simulink model "TBRe19_ECU_SequentialTests"  (R2017b)
settings: Solver=FixedStepDiscrete  StartTime=0.0  StopTime=inf  FixedStep=0.0001  RelTol=1e-3
PostLoadFcn:
  | model_init();
libraries: simulink x28
(part 19 of 22)

== system TBRe19_ECU_SequentialTests/RTDandStateMachine/Comms_And_Data_Acquisition_Layer/Hardwired_Inputs_2019/BMS ==
  DigitalInput1 : S-Function  FunctionName=NsiIo_DigitalInput  Parameters=channel,is_trigger,typeof_trigger,is_wakeup,wakeup_level  SFunctionDeploymentMode=off  EnableBusSupport=off  mask(MUXlink I/O Digital Input){channel=16, is_trigger=off, typeof_trigger=Either, is_wakeup=off, wakeup_level=Low level}
      mask prompts: channel "Channel ?"; is_trigger "Trigger ?"; typeof_trigger "Type of Trigger ?"; is_wakeup "Wake-up ?"; wakeup_level "Wake-up level ?"
      mask help: Read digital input from I/O channel.
      mask init:
      | NsiIo_DigitalInput_InitializationFcn();
      settings: OpenFcn=NsiIo_DigitalInput_OpenFcn();
      mask Help:
      | eval('block=get_param(gcb, ''RTWdata'');')
      | web([docroot '\toolbox\MUXlink\html\blocks/' block.MUXlink_BlockType '.html'])
      mask Callback channel: NsiIo_DigitalInput_ApplyFcn(1);
      mask Callback is_trigger: NsiIo_DigitalInput_ApplyFcn(2);
      mask TypeOptions typeof_trigger: Rising | Falling | Either
      mask Callback typeof_trigger: NsiIo_DigitalInput_ApplyFcn(3);
      mask Callback is_wakeup: NsiIo_DigitalInput_ApplyFcn(4);
      mask TypeOptions wakeup_level: Low level | High level
      mask Callback wakeup_level: NsiIo_DigitalInput_ApplyFcn(5);
      mask Display: image(imread('nsi.bmp'));text(0.5, 0.2, 'DigitalInput_16', 'horizontalAlignment', 'center', 'verticalAlignment', 'base');plot([0.05 0.05 0.05 0.05 0.05 0.05 0.05 0.05 0.05 0.05]);port_label('output', 1, 'Battery : H2');
  DigitalInput2 : S-Function  FunctionName=NsiIo_DigitalInput  Parameters=channel,is_trigger,typeof_trigger,is_wakeup,wakeup_level  SFunctionDeploymentMode=off  EnableBusSupport=off  mask(MUXlink I/O Digital Input){channel=17, is_trigger=off, typeof_trigger=Either, is_wakeup=off, wakeup_level=Low level}
      mask prompts: channel "Channel ?"; is_trigger "Trigger ?"; typeof_trigger "Type of Trigger ?"; is_wakeup "Wake-up ?"; wakeup_level "Wake-up level ?"
      mask help: Read digital input from I/O channel.
      mask init:
      | NsiIo_DigitalInput_InitializationFcn();
      settings: OpenFcn=NsiIo_DigitalInput_OpenFcn();
      mask Help:
      | eval('block=get_param(gcb, ''RTWdata'');')
      | web([docroot '\toolbox\MUXlink\html\blocks/' block.MUXlink_BlockType '.html'])
      mask Callback channel: NsiIo_DigitalInput_ApplyFcn(1);
      mask Callback is_trigger: NsiIo_DigitalInput_ApplyFcn(2);
      mask TypeOptions typeof_trigger: Rising | Falling | Either
      mask Callback typeof_trigger: NsiIo_DigitalInput_ApplyFcn(3);
      mask Callback is_wakeup: NsiIo_DigitalInput_ApplyFcn(4);
      mask TypeOptions wakeup_level: Low level | High level
      mask Callback wakeup_level: NsiIo_DigitalInput_ApplyFcn(5);
      mask Display: image(imread('nsi.bmp'));text(0.5, 0.2, 'DigitalInput_17', 'horizontalAlignment', 'center', 'verticalAlignment', 'base');plot([0.05 0.05 0.05 0.05 0.05 0.05 0.05 0.05 0.05 0.05]);port_label('output', 1, 'Battery : H3');
  DigitalInput6 : S-Function  FunctionName=NsiIo_DigitalInput  Parameters=channel,is_trigger,typeof_trigger,is_wakeup,wakeup_level  SFunctionDeploymentMode=off  EnableBusSupport=off  mask(MUXlink I/O Digital Input){channel=18, is_trigger=off, typeof_trigger=Either, is_wakeup=off, wakeup_level=Low level}
      mask prompts: channel "Channel ?"; is_trigger "Trigger ?"; typeof_trigger "Type of Trigger ?"; is_wakeup "Wake-up ?"; wakeup_level "Wake-up level ?"
      mask help: Read digital input from I/O channel.
      mask init:
      | NsiIo_DigitalInput_InitializationFcn();
      settings: OpenFcn=NsiIo_DigitalInput_OpenFcn();
      mask Help:
      | eval('block=get_param(gcb, ''RTWdata'');')
      | web([docroot '\toolbox\MUXlink\html\blocks/' block.MUXlink_BlockType '.html'])
      mask Callback channel: NsiIo_DigitalInput_ApplyFcn(1);
      mask Callback is_trigger: NsiIo_DigitalInput_ApplyFcn(2);
      mask TypeOptions typeof_trigger: Rising | Falling | Either
      mask Callback typeof_trigger: NsiIo_DigitalInput_ApplyFcn(3);
      mask Callback is_wakeup: NsiIo_DigitalInput_ApplyFcn(4);
      mask TypeOptions wakeup_level: Low level | High level
      mask Callback wakeup_level: NsiIo_DigitalInput_ApplyFcn(5);
      mask Display: image(imread('nsi.bmp'));text(0.5, 0.2, 'DigitalInput_18', 'horizontalAlignment', 'center', 'verticalAlignment', 'base');plot([0.05 0.05 0.05 0.05 0.05 0.05 0.05 0.05 0.05 0.05]);port_label('output', 1, 'Battery : H4');
  BMS_Multi1 : Outport
  BMS_Multi2 : Outport  Port=2
  BMS_ChargeEnable : Outport  Port=3
  wires:
  DigitalInput6/1 -> BMS_Multi1/1  "BMS_Multi1"
  DigitalInput2/1 -> BMS_ChargeEnable/1  "BMS_ChargeEnable"
  DigitalInput1/1 -> BMS_Multi2/1  "BMS_Multi2"

== system TBRe19_ECU_SequentialTests/RTDandStateMachine/Comms_And_Data_Acquisition_Layer/Hardwired_Inputs_2019/Buttons ==
  DigitalInput1 : S-Function  FunctionName=NsiIo_DigitalInput  Parameters=channel,is_trigger,typeof_trigger,is_wakeup,wakeup_level  SFunctionDeploymentMode=off  EnableBusSupport=off  mask(MUXlink I/O Digital Input){channel=5, is_trigger=off, typeof_trigger=Either, is_wakeup=off, wakeup_level=Low level}
      mask prompts: channel "Channel ?"; is_trigger "Trigger ?"; typeof_trigger "Type of Trigger ?"; is_wakeup "Wake-up ?"; wakeup_level "Wake-up level ?"
      mask help: Read digital input from I/O channel.
      mask init:
      | NsiIo_DigitalInput_InitializationFcn();
      settings: OpenFcn=NsiIo_DigitalInput_OpenFcn();
      mask Help:
      | eval('block=get_param(gcb, ''RTWdata'');')
      | web([docroot '\toolbox\MUXlink\html\blocks/' block.MUXlink_BlockType '.html'])
      mask Callback channel: NsiIo_DigitalInput_ApplyFcn(1);
      mask Callback is_trigger: NsiIo_DigitalInput_ApplyFcn(2);
      mask TypeOptions typeof_trigger: Rising | Falling | Either
      mask Callback typeof_trigger: NsiIo_DigitalInput_ApplyFcn(3);
      mask Callback is_wakeup: NsiIo_DigitalInput_ApplyFcn(4);
      mask TypeOptions wakeup_level: Low level | High level
      mask Callback wakeup_level: NsiIo_DigitalInput_ApplyFcn(5);
      mask Display: image(imread('nsi.bmp'));text(0.5, 0.2, 'DigitalInput_5', 'horizontalAlignment', 'center', 'verticalAlignment', 'base');plot([0.05 0.05 0.05 0.05 0.05 0.05 0.05 0.05 0.05 0.05]);port_label('output', 1, 'Ground : B1');
  DigitalInput2 : S-Function  FunctionName=NsiIo_DigitalInput  Parameters=channel,is_trigger,typeof_trigger,is_wakeup,wakeup_level  SFunctionDeploymentMode=off  EnableBusSupport=off  mask(MUXlink I/O Digital Input){channel=8, is_trigger=off, typeof_trigger=Either, is_wakeup=off, wakeup_level=Low level}
      mask prompts: channel "Channel ?"; is_trigger "Trigger ?"; typeof_trigger "Type of Trigger ?"; is_wakeup "Wake-up ?"; wakeup_level "Wake-up level ?"
      mask help: Read digital input from I/O channel.
      mask init:
      | NsiIo_DigitalInput_InitializationFcn();
      settings: OpenFcn=NsiIo_DigitalInput_OpenFcn();
      mask Help:
      | eval('block=get_param(gcb, ''RTWdata'');')
      | web([docroot '\toolbox\MUXlink\html\blocks/' block.MUXlink_BlockType '.html'])
      mask Callback channel: NsiIo_DigitalInput_ApplyFcn(1);
      mask Callback is_trigger: NsiIo_DigitalInput_ApplyFcn(2);
      mask TypeOptions typeof_trigger: Rising | Falling | Either
      mask Callback typeof_trigger: NsiIo_DigitalInput_ApplyFcn(3);
      mask Callback is_wakeup: NsiIo_DigitalInput_ApplyFcn(4);
      mask TypeOptions wakeup_level: Low level | High level
      mask Callback wakeup_level: NsiIo_DigitalInput_ApplyFcn(5);
      mask Display: image(imread('nsi.bmp'));text(0.5, 0.2, 'DigitalInput_8', 'horizontalAlignment', 'center', 'verticalAlignment', 'base');plot([0.05 0.05 0.05 0.05 0.05 0.05 0.05 0.05 0.05 0.05]);port_label('output', 1, 'Ground : B4');
  DigitalInput3 : S-Function  FunctionName=NsiIo_DigitalInput  Parameters=channel,is_trigger,typeof_trigger,is_wakeup,wakeup_level  SFunctionDeploymentMode=off  EnableBusSupport=off  mask(MUXlink I/O Digital Input){channel=6, is_trigger=off, typeof_trigger=Either, is_wakeup=off, wakeup_level=Low level}
      mask prompts: channel "Channel ?"; is_trigger "Trigger ?"; typeof_trigger "Type of Trigger ?"; is_wakeup "Wake-up ?"; wakeup_level "Wake-up level ?"
      mask help: Read digital input from I/O channel.
      mask init:
      | NsiIo_DigitalInput_InitializationFcn();
      settings: OpenFcn=NsiIo_DigitalInput_OpenFcn();
      mask Help:
      | eval('block=get_param(gcb, ''RTWdata'');')
      | web([docroot '\toolbox\MUXlink\html\blocks/' block.MUXlink_BlockType '.html'])
      mask Callback channel: NsiIo_DigitalInput_ApplyFcn(1);
      mask Callback is_trigger: NsiIo_DigitalInput_ApplyFcn(2);
      mask TypeOptions typeof_trigger: Rising | Falling | Either
      mask Callback typeof_trigger: NsiIo_DigitalInput_ApplyFcn(3);
      mask Callback is_wakeup: NsiIo_DigitalInput_ApplyFcn(4);
      mask TypeOptions wakeup_level: Low level | High level
      mask Callback wakeup_level: NsiIo_DigitalInput_ApplyFcn(5);
      mask Display: image(imread('nsi.bmp'));text(0.5, 0.2, 'DigitalInput_6', 'horizontalAlignment', 'center', 'verticalAlignment', 'base');plot([0.05 0.05 0.05 0.05 0.05 0.05 0.05 0.05 0.05 0.05]);port_label('output', 1, 'Ground : B2');
  DigitalInput4 : S-Function  FunctionName=NsiIo_DigitalInput  Parameters=channel,is_trigger,typeof_trigger,is_wakeup,wakeup_level  SFunctionDeploymentMode=off  EnableBusSupport=off  mask(MUXlink I/O Digital Input){channel=7, is_trigger=off, typeof_trigger=Either, is_wakeup=off, wakeup_level=Low level}
      mask prompts: channel "Channel ?"; is_trigger "Trigger ?"; typeof_trigger "Type of Trigger ?"; is_wakeup "Wake-up ?"; wakeup_level "Wake-up level ?"
      mask help: Read digital input from I/O channel.
      mask init:
      | NsiIo_DigitalInput_InitializationFcn();
      settings: OpenFcn=NsiIo_DigitalInput_OpenFcn();
      mask Help:
      | eval('block=get_param(gcb, ''RTWdata'');')
      | web([docroot '\toolbox\MUXlink\html\blocks/' block.MUXlink_BlockType '.html'])
      mask Callback channel: NsiIo_DigitalInput_ApplyFcn(1);
      mask Callback is_trigger: NsiIo_DigitalInput_ApplyFcn(2);
      mask TypeOptions typeof_trigger: Rising | Falling | Either
      mask Callback typeof_trigger: NsiIo_DigitalInput_ApplyFcn(3);
      mask Callback is_wakeup: NsiIo_DigitalInput_ApplyFcn(4);
      mask TypeOptions wakeup_level: Low level | High level
      mask Callback wakeup_level: NsiIo_DigitalInput_ApplyFcn(5);
      mask Display: image(imread('nsi.bmp'));text(0.5, 0.2, 'DigitalInput_7', 'horizontalAlignment', 'center', 'verticalAlignment', 'base');plot([0.05 0.05 0.05 0.05 0.05 0.05 0.05 0.05 0.05 0.05]);port_label('output', 1, 'Ground : B3');
  DigitalInput5 : S-Function  FunctionName=NsiIo_DigitalInput  Parameters=channel,is_trigger,typeof_trigger,is_wakeup,wakeup_level  SFunctionDeploymentMode=off  EnableBusSupport=off  mask(MUXlink I/O Digital Input){channel=9, is_trigger=off, typeof_trigger=Either, is_wakeup=off, wakeup_level=Low level}
      mask prompts: channel "Channel ?"; is_trigger "Trigger ?"; typeof_trigger "Type of Trigger ?"; is_wakeup "Wake-up ?"; wakeup_level "Wake-up level ?"
      mask help: Read digital input from I/O channel.
      mask init:
      | NsiIo_DigitalInput_InitializationFcn();
      settings: OpenFcn=NsiIo_DigitalInput_OpenFcn();
      mask Help:
      | eval('block=get_param(gcb, ''RTWdata'');')
      | web([docroot '\toolbox\MUXlink\html\blocks/' block.MUXlink_BlockType '.html'])
      mask Callback channel: NsiIo_DigitalInput_ApplyFcn(1);
      mask Callback is_trigger: NsiIo_DigitalInput_ApplyFcn(2);
      mask TypeOptions typeof_trigger: Rising | Falling | Either
      mask Callback typeof_trigger: NsiIo_DigitalInput_ApplyFcn(3);
      mask Callback is_wakeup: NsiIo_DigitalInput_ApplyFcn(4);
      mask TypeOptions wakeup_level: Low level | High level
      mask Callback wakeup_level: NsiIo_DigitalInput_ApplyFcn(5);
      mask Display: image(imread('nsi.bmp'));text(0.5, 0.2, 'DigitalInput_9', 'horizontalAlignment', 'center', 'verticalAlignment', 'base');plot([0.05 0.05 0.05 0.05 0.05 0.05 0.05 0.05 0.05 0.05]);port_label('output', 1, 'Battery : C1');
  DigitalInput6 : S-Function  FunctionName=NsiIo_DigitalInput  Parameters=channel,is_trigger,typeof_trigger,is_wakeup,wakeup_level  SFunctionDeploymentMode=off  EnableBusSupport=off  mask(MUXlink I/O Digital Input){channel=10, is_trigger=off, typeof_trigger=Either, is_wakeup=off, wakeup_level=Low level}
      mask prompts: channel "Channel ?"; is_trigger "Trigger ?"; typeof_trigger "Type of Trigger ?"; is_wakeup "Wake-up ?"; wakeup_level "Wake-up level ?"
      mask help: Read digital input from I/O channel.
      mask init:
      | NsiIo_DigitalInput_InitializationFcn();
      settings: OpenFcn=NsiIo_DigitalInput_OpenFcn();
      mask Help:
      | eval('block=get_param(gcb, ''RTWdata'');')
      | web([docroot '\toolbox\MUXlink\html\blocks/' block.MUXlink_BlockType '.html'])
      mask Callback channel: NsiIo_DigitalInput_ApplyFcn(1);
      mask Callback is_trigger: NsiIo_DigitalInput_ApplyFcn(2);
      mask TypeOptions typeof_trigger: Rising | Falling | Either
      mask Callback typeof_trigger: NsiIo_DigitalInput_ApplyFcn(3);
      mask Callback is_wakeup: NsiIo_DigitalInput_ApplyFcn(4);
      mask TypeOptions wakeup_level: Low level | High level
      mask Callback wakeup_level: NsiIo_DigitalInput_ApplyFcn(5);
      mask Display: image(imread('nsi.bmp'));text(0.5, 0.2, 'DigitalInput_10', 'horizontalAlignment', 'center', 'verticalAlignment', 'base');plot([0.05 0.05 0.05 0.05 0.05 0.05 0.05 0.05 0.05 0.05]);port_label('output', 1, 'Battery : C2');
  btnRTD_Input : Outport
  btnX_Input : Outport  Port=2
  btnY_Input : Outport  Port=3
  btnZ_Input : Outport  Port=4
  btnPumpFan_Input : Outport  Port=5
  btnAccyFan_Input : Outport  Port=6
  wires:
  DigitalInput1/1 -> btnRTD_Input/1  "btnRTD_Input"
  DigitalInput4/1 -> btnY_Input/1  "btnY_Input"
  DigitalInput3/1 -> btnX_Input/1  "btnX_Input"
  DigitalInput2/1 -> btnZ_Input/1  "btnZ_Input"
  DigitalInput5/1 -> btnPumpFan_Input/1  "btnPumpFan_Input"
  DigitalInput6/1 -> btnAccyFan_Input/1  "btnAccyFan_Input"

== system TBRe19_ECU_SequentialTests/RTDandStateMachine/Comms_And_Data_Acquisition_Layer/Hardwired_Inputs_2019/Pedal_Box ==
  AnalogInput1 : S-Function  FunctionName=NsiIo_AnalogInput  Parameters=channel  SFunctionDeploymentMode=off  EnableBusSupport=off  mask(MUXlink I/O Analog Input){channel=1, RANGE=0 / 20 Volts}
      mask prompts: channel "Channel ?"; RANGE "Plage de mesure"
      mask help: This block interface the 8 Analog Inputs. Channels 1 to 4 are 0/10V, and the channels 5 to 8 are0/20V. Voltage input is read in mV
      mask init:
      | NsiIo_AnalogInput_InitializationFcn();
      settings: OpenFcn=NsiIo_AnalogInput_OpenFcn();
      mask Help:
      | eval('block=get_param(gcb, ''RTWdata'');')
      | web([docroot '\toolbox\MUXlink\html\blocks/' block.MUXlink_BlockType '.html'])
      mask Callback channel: NsiIo_AnalogInput_ApplyFcn();
      mask Callback RANGE: NsiIo_AnalogInput_ApplyFcn();
      mask Display: image(imread('nsi.bmp'));text(0.5, 0.2, 'AnalogInput_1\n\n0 / 20 Volts', 'horizontalAlignment', 'center', 'verticalAlignment', 'base');plot([0.05 0.05 0.05 0.05 0.05 0.05 0.05 0.05 0.05 0.05]);port_label('output', 1, 'B1');
  AnalogInput2 : S-Function  FunctionName=NsiIo_AnalogInput  Parameters=channel  SFunctionDeploymentMode=off  EnableBusSupport=off  mask(MUXlink I/O Analog Input){channel=3, RANGE=0 / 20 Volts}
      mask prompts: channel "Channel ?"; RANGE "Plage de mesure"
      mask help: This block interface one of the 8 Analog Inputs. The analog inputs must be in the 0/20V range. Voltage output port provide a value in mV
      mask init:
      | NsiIo_AnalogInput_InitializationFcn();
      settings: OpenFcn=NsiIo_AnalogInput_OpenFcn();
      mask Help:
      | eval('block=get_param(gcb, ''RTWdata'');')
      | web([docroot '\toolbox\MUXlink\html\blocks/' block.MUXlink_BlockType '.html'])
      mask Callback channel: NsiIo_AnalogInput_ApplyFcn();
      mask Callback RANGE: NsiIo_AnalogInput_ApplyFcn();
      mask Display: image(imread('nsi.bmp'));text(0.5, 0.2, 'AnalogInput_3\n\n0 / 20 Volts', 'horizontalAlignment', 'center', 'verticalAlignment', 'base');plot([0.05 0.05 0.05 0.05 0.05 0.05 0.05 0.05 0.05 0.05]);port_label('output', 1, 'B3');
  AnalogInput3 : S-Function  FunctionName=NsiIo_AnalogInput  Parameters=channel  SFunctionDeploymentMode=off  EnableBusSupport=off  mask(MUXlink I/O Analog Input){channel=4, RANGE=0 / 20 Volts}
      mask prompts: channel "Channel ?"; RANGE "Plage de mesure"
      mask help: This block interface one of the 8 Analog Inputs. The analog inputs must be in the 0/20V range. Voltage output port provide a value in mV
      mask init:
      | NsiIo_AnalogInput_InitializationFcn();
      settings: OpenFcn=NsiIo_AnalogInput_OpenFcn();
      mask Help:
      | eval('block=get_param(gcb, ''RTWdata'');')
      | web([docroot '\toolbox\MUXlink\html\blocks/' block.MUXlink_BlockType '.html'])
      mask Callback channel: NsiIo_AnalogInput_ApplyFcn();
      mask Callback RANGE: NsiIo_AnalogInput_ApplyFcn();
      mask Display: image(imread('nsi.bmp'));text(0.5, 0.2, 'AnalogInput_4\n\n0 / 20 Volts', 'horizontalAlignment', 'center', 'verticalAlignment', 'base');plot([0.05 0.05 0.05 0.05 0.05 0.05 0.05 0.05 0.05 0.05]);port_label('output', 1, 'B4');
  AnalogInput6 : S-Function  FunctionName=NsiIo_AnalogInput  Parameters=channel  SFunctionDeploymentMode=off  EnableBusSupport=off  mask(MUXlink I/O Analog Input){channel=2, RANGE=0 / 20 Volts}
      mask prompts: channel "Channel ?"; RANGE "Plage de mesure"
      mask help: This block interface one of the 8 Analog Inputs. The analog inputs must be in the 0/20V range. Voltage output port provide a value in mV
      mask init:
      | NsiIo_AnalogInput_InitializationFcn();
      settings: OpenFcn=NsiIo_AnalogInput_OpenFcn();
      mask Help:
      | eval('block=get_param(gcb, ''RTWdata'');')
      | web([docroot '\toolbox\MUXlink\html\blocks/' block.MUXlink_BlockType '.html'])
      mask Callback channel: NsiIo_AnalogInput_ApplyFcn();
      mask Callback RANGE: NsiIo_AnalogInput_ApplyFcn();
      mask Display: image(imread('nsi.bmp'));text(0.5, 0.2, 'AnalogInput_2\n\n0 / 20 Volts', 'horizontalAlignment', 'center', 'verticalAlignment', 'base');plot([0.05 0.05 0.05 0.05 0.05 0.05 0.05 0.05 0.05 0.05]);port_label('output', 1, 'B2');
  AnalogInput7 : S-Function  FunctionName=NsiIo_AnalogInput  Parameters=channel  SFunctionDeploymentMode=off  EnableBusSupport=off  mask(MUXlink I/O Analog Input){channel=6, RANGE=0 / 20 Volts}
      mask prompts: channel "Channel ?"; RANGE "Plage de mesure"
      mask help: This block interface one of the 8 Analog Inputs. The analog inputs must be in the 0/20V range. Voltage output port provide a value in mV
      mask init:
      | NsiIo_AnalogInput_InitializationFcn();
      settings: OpenFcn=NsiIo_AnalogInput_OpenFcn();
      mask Help:
      | eval('block=get_param(gcb, ''RTWdata'');')
      | web([docroot '\toolbox\MUXlink\html\blocks/' block.MUXlink_BlockType '.html'])
      mask Callback channel: NsiIo_AnalogInput_ApplyFcn();
      mask Callback RANGE: NsiIo_AnalogInput_ApplyFcn();
      mask Display: image(imread('nsi.bmp'));text(0.5, 0.2, 'AnalogInput_6\n\n0 / 20 Volts', 'horizontalAlignment', 'center', 'verticalAlignment', 'base');plot([0.05 0.05 0.05 0.05 0.05 0.05 0.05 0.05 0.05 0.05]);port_label('output', 1, 'C4');
  Throttle1_Voltage : Outport
  Throttle2_Voltage : Outport  Port=2
  Brake_Voltage : Outport  Port=3
  Brake1_Pressure : Outport  Port=4
  Brake2_Pressure : Outport  Port=5
  wires:
  AnalogInput6/1 -> Throttle2_Voltage/1  "Throttle2_Voltage"
  AnalogInput1/1 -> Throttle1_Voltage/1  "Throttle1_Voltage"
  AnalogInput7/1 -> Brake_Voltage/1  "Brake_POT"
  AnalogInput2/1 -> Brake1_Pressure/1  "Brake1_Pressure"
  AnalogInput3/1 -> Brake2_Pressure/1  "Brake2_Pressure"

== system TBRe19_ECU_SequentialTests/RTDandStateMachine/Pre_Processing_Layer/Pedal_Box/APPS and BP Plausibility ==
  note: Invert the logic so that if error is active, throttle gets multiplied by zero
  note: This block outputs the previous state from previous sample
  note: Note: This is needed by rules - including specified percentages
  note: If brake is above 20% AND accelerator is above 25%, then hold the error on until throttle is less than 5%
  note: If accelerator and brake pedal are pressed at the same time, then wait for both pedals to return to zero before sending further torque requests
  note: function [Throttle_Percentage, APPS_BP_Implausibility] = APPS_BP_Plausibility_Check(Throttle_In, Brake_In, APPS_BP_Implausibility_Prv)
      | %Plausibility check on both throttle and brake
      |
      | %Implausible case: when both brake and throttle applied
      | if (Brake_In >=20 && Throttle_In > 25)
      |     APPS_BP_Implausibility = true;
      |     Throttle_Percentage =uint8(0);
      |
      | %Implausible case: when brake pressed but throttle still not below 5%
      | elseif (APPS_BP_Implausibility_Prv && Throttle_In > 5)
      |     APPS_BP_Implausibility = true;
      |     Throttle_Percentage =uint8(0);
      |
      | %Plausible case, throttle goes below 5%
      | elseif (APPS_BP_Implausibility_Prv && Throttle_In < 5)
      |     APPS_BP_Implausibility = false;
      |     Throttle_Percentage =uint8(Throttle_In);
      |
      | %Plausible case, normal operation
      | else
      |     APPS_BP_Implausibility = false;
      |     Throttle_Percentage =uint8(Throttle_In);
      | end
  Throttle_In : Inport
  Brake_% : Inport  Port=2
  Constant : Constant  Value=20
  Constant1 : Constant  Value=25
  Constant2 : Constant  Value=5
  Logical Operator : Logic  AllPortsSameDT=off  OutDataTypeStr=boolean
  Logical Operator1 : Logic  AllPortsSameDT=off  OutDataTypeStr=boolean
  Logical Operator2 : Logic  Operator=OR  AllPortsSameDT=off  OutDataTypeStr=boolean
  Logical Operator3 : Logic  Operator=NOT  Inputs=1  AllPortsSameDT=off  OutDataTypeStr=boolean
  Product : Product  OutDataTypeStr=uint8
  Relational Operator : RelationalOperator  OutDataTypeStr=boolean  RndMeth=Simplest
  Relational Operator1 : RelationalOperator  Operator=>  OutDataTypeStr=boolean  RndMeth=Simplest
  Relational Operator2 : RelationalOperator  Operator=>  OutDataTypeStr=boolean  RndMeth=Simplest
  prv_APPS_BP1 : Delay  DelayLength=1  InitialCondition=0
  Throttle_% : Outport
  APPS_BP_Implausibility : Outport  Port=2
  wires:
  Brake_%/1 -> Relational Operator/1
  Constant/1 -> Relational Operator/2
  Constant1/1 -> Relational Operator1/2
  Constant2/1 -> Relational Operator2/2
  Throttle_In/1 -> Product/2, Relational Operator2/1, Relational Operator1/1
  prv_APPS_BP1/1 -> Logical Operator1/2
  Relational Operator2/1 -> Logical Operator1/1
  Relational Operator/1 -> Logical Operator/1
  Relational Operator1/1 -> Logical Operator/2
  Logical Operator2/1 -> APPS_BP_Implausibility/1, Logical Operator3/1, prv_APPS_BP1/1
  Logical Operator1/1 -> Logical Operator2/2
  Logical Operator/1 -> Logical Operator2/1
  Product/1 -> Throttle_%/1
  Logical Operator3/1 -> Product/1

== system TBRe19_ECU_SequentialTests/RTDandStateMachine/Pre_Processing_Layer/Pedal_Box/APPS_Implausibility_Check ==
  note: This sets torque to zero if APPS implausibility happens
  note: Send to CAN bus
  note: Note: 100ms is measured using 10 delays. As task runs every 10ms, 10 delays will result in a 100ms delay
  note: If the error happens continuosly for 100ms then the throttle output should be set to zero
  note: Check to see if Throttle2 is within the range of Throttle1 +/- 15%
  note: 15% is defined in rules
  note: Remember to change to "min"
      | when we have both sensors installed
  note: function [APPS_Implausbility, Throttle_Percentage] = APPS_Implausibility_Check(Pedal_Sensor_Fail, Throttle1_Per, Throttle2_Per)
      | %Limit generation for comparison
      | Upper_Limit = Throttle1_Per+15;
      | Lower_Limit = Throttle1_Per-15;
      |
      | %Passes one throttle if in range and no pedal sensor errors
      | if ((Lower_Limit <= Throttle2_Per) && (Throttle2_Per <= Upper_Limit)&& Pedal_Sensor_Fail == 0)
      |     Throttle_Percentage = uint8(max(Throttle1_Per, Throttle2_Per));
      |     APPS_Implausbility = false;
      | %All other conditions result in no throttle being applied
      | else
      |     Throttle_Percentage = uint8(0);
      |     APPS_Implausbility = true;
      | end
      |
      | end
  Throttle1_Per : Inport
  Throttle2_Per : Inport  Port=2
  Constant : Constant  Value=15
  Data Type Conversion : DataTypeConversion  OutDataTypeStr=int8
  Logical Operator : Logic  Operator=OR  AllPortsSameDT=off  OutDataTypeStr=boolean
  Logical Operator3 : Logic  Operator=NOT  Inputs=1  AllPortsSameDT=off  OutDataTypeStr=boolean
  LowerLinit : Sum  Inputs=-+
  MinMax : MinMax  Function=max  Inputs=2
  Product : Product
  Product of Elements : Product  Inputs=*
  Relational Operator : RelationalOperator  OutDataTypeStr=boolean  RndMeth=Simplest
  Relational Operator1 : RelationalOperator  Operator=<=  OutDataTypeStr=boolean  RndMeth=Simplest
  Tapped Delay : simulink/Discrete/Tapped Delay  vinit=0  samptime=-1  NumDelays=10  DelayOrder=Oldest  includeCurrent=off
  UpperLinit : Sum
  APPS_Implausibility : Outport
  Throttle_% : Outport  Port=2
  wires:
  Throttle1_Per/1 -> MinMax/1, UpperLinit/1, LowerLinit/2
  Throttle2_Per/1 -> MinMax/2, Relational Operator1/1, Relational Operator/1
  Logical Operator/1 -> Tapped Delay/1  "APPS_Implausibility"
  Constant/1 -> UpperLinit/2, LowerLinit/1
  UpperLinit/1 -> Relational Operator/2
  LowerLinit/1 -> Relational Operator1/2
  Relational Operator/1 -> Logical Operator/1
  Relational Operator1/1 -> Logical Operator/2
  Logical Operator3/1 -> Data Type Conversion/1
  Data Type Conversion/1 -> Product/2
  MinMax/1 -> Throttle_%/1
  Tapped Delay/1 -> Product of Elements/1
  Product of Elements/1 -> APPS_Implausibility/1, Logical Operator3/1

== system TBRe19_ECU_SequentialTests/RTDandStateMachine/Pre_Processing_Layer/Pedal_Box/BPPS_Implausibility_Check ==
  note: Note: Not needed for rules
  note: Output to CAN
  note: function [APPS_Implausbility, Throttle_Percentage] = APPS_Implausibility_Check(Pedal_Sensor_Fail, Throttle1_Per, Throttle2_Per)
      | %Limit generation for comparison
      | Upper_Limit = Throttle1_Per+15;
      | Lower_Limit = Throttle1_Per-15;
      |
      | %Passes one throttle if in range and no pedal sensor errors
      | if ((Lower_Limit <= Throttle2_Per) && (Throttle2_Per <= Upper_Limit)&& Pedal_Sensor_Fail == 0)
      |     Throttle_Percentage = uint8(max(Throttle1_Per, Throttle2_Per));
      |     APPS_Implausbility = false;
      | %All other conditions result in no throttle being applied
      | else
      |     Throttle_Percentage = uint8(0);
      |     APPS_Implausbility = true;
      | end
      |
      | end
  note: If the error happens continuosly for 100ms then the throttle output should be set to zero
  note: Note: 100ms is measured using 10 delays. As task runs every 10ms, 10 delays will result in a 100ms delay
  Brake1_Per : Inport
  Brake2_Per : Inport  Port=2
  Constant : Constant  Value=15
  Logical Operator : Logic  Operator=OR  AllPortsSameDT=off  OutDataTypeStr=boolean
  LowerLinit : Sum  Inputs=-+
  MinMax : MinMax  Inputs=2
  Product of Elements : Product  Inputs=*
  Relational Operator : RelationalOperator  OutDataTypeStr=boolean  RndMeth=Simplest
  Relational Operator1 : RelationalOperator  Operator=<=  OutDataTypeStr=boolean  RndMeth=Simplest
  Tapped Delay : simulink/Discrete/Tapped Delay  vinit=0  samptime=-1  NumDelays=10  DelayOrder=Oldest  includeCurrent=off
  UpperLinit : Sum
  Brake_% : Outport
  BPPS_Implausibility : Outport  Port=2
  wires:
  Brake1_Per/1 -> MinMax/1, UpperLinit/1, LowerLinit/2
  Brake2_Per/1 -> MinMax/2, Relational Operator1/1, Relational Operator/1
  Logical Operator/1 -> Tapped Delay/1  "APPS_Implausibility"
  Constant/1 -> UpperLinit/2, LowerLinit/1
  UpperLinit/1 -> Relational Operator/2
  LowerLinit/1 -> Relational Operator1/2
  Relational Operator/1 -> Logical Operator/1
  Relational Operator1/1 -> Logical Operator/2
  Tapped Delay/1 -> Product of Elements/1
  Product of Elements/1 -> BPPS_Implausibility/1
  MinMax/1 -> Brake_%/1

== system TBRe19_ECU_SequentialTests/RTDandStateMachine/Pre_Processing_Layer/Pedal_Box/Sensor Plausibility ==
  note: Check if the readings from the sensors are outside expected range
      | e.g. If a 5V sensor is giving a reading of 12V
      |
      | Note: Not needed for rules
  <Throttle1_Voltage> : Inport
  <Throttle2_Voltage> : Inport  Port=2
  <Brake_Voltage> : Inport  Port=3
  <Brake_Voltage>1 : Inport  Port=4
  <Brake_Voltage>2 : Inport  Port=5
  Sensor_Diag : MATLAB Function  TreatAsAtomicUnit=on
  Pedal_Sensor_Fail : Outport
  TV1_Out : Outport  Port=2
  TV2_Out : Outport  Port=3
  BVPot_Out : Outport  Port=4
  BV1_Out : Outport  Port=5
  BV1_Out1 : Outport  Port=6
  wires:
  <Throttle1_Voltage>/1 -> Sensor_Diag/1(TV_1)
  <Throttle2_Voltage>/1 -> Sensor_Diag/2(TV_2)
  <Brake_Voltage>/1 -> Sensor_Diag/3(BV_POT)
  Sensor_Diag/1(Pedal_Sensor_Fail) -> Pedal_Sensor_Fail/1
  Sensor_Diag/2(TV1_Out) -> TV1_Out/1
  Sensor_Diag/3(TV2_Out) -> TV2_Out/1
  Sensor_Diag/4(BVPot_Out) -> BVPot_Out/1
  <Brake_Voltage>1/1 -> Sensor_Diag/4(BV_1)
  <Brake_Voltage>2/1 -> Sensor_Diag/5(BV_2)
  Sensor_Diag/5(BV1_Out) -> BV1_Out/1
  Sensor_Diag/6(BV2_Out) -> BV1_Out1/1
